simulink model "cartpole"  (R2016a)
settings: Solver=ode23s  StartTime=0.0  StopTime=90  RelTol=1e-3
values from neighbouring files (symbols this model uses):
  g = 9.81    [cartPole.mat]
  K = lqr(A,B,Q,R)    [KDC_HW2_Problem4_LQR.m]    (also in cartPole.mat = [143.360926463 -1 35.2365734727 -11.2706480711])
  kd = 0.1    [cartPole.mat]
  ke = 2    [cartPole.mat]
  kp = 0.1    [cartPole.mat]
  l = 1    [cartPole.mat]
  mc = 1    [cartPole.mat]
  mp = 0.1    [cartPole.mat]
libraries: mblibv1 x11, simulink x1
settings Model: Creator=Bradley Factor  LastModifiedBy=Bradley Factor
settings SolverCC: MaxConsecutiveMinStep=100
settings SimMechanicsCC: VisDuringSimulation=on

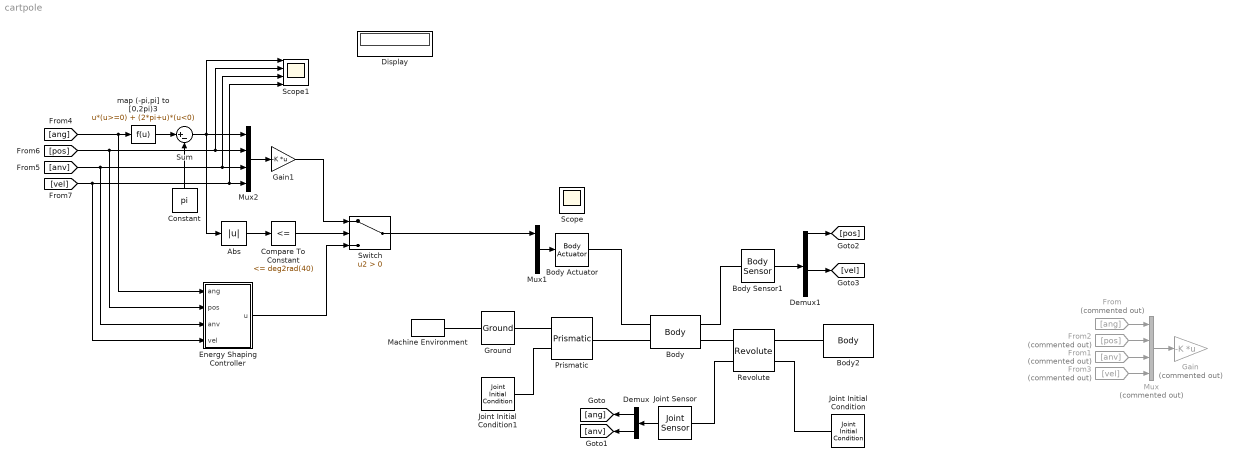
== system cartpole ==
  Abs : Abs
  Body : mblibv1/Bodies/Body  LConnTagsString=CS4|CS1  RConnTagsString=CG|CS3  UpdateFromCAD=off  DialogClass=MechanicalBodyBlock  Mass=1  MassUnits=kg  InertiaUnits=kg*m^2  Inertia=eye(3)  Shape=Cylinder  ShapeDims=[1 1]  ShapeUnits=m  ShapeUse=false  Density=1  DensityUnits=kg/m^3  DensityUse=false  GraphicsMode=MACHINE_DEFAULT  BodyColorSelMode=MACHINE_DEFAULT  BodyColor=[1 0 0]  AttachedToCS=CG  CG=Right$CG$[0.25 0 0]$CS1$CS1$m$[0 0 0]$Euler X-Y-Z$deg$WORLD$true$none  WorkingFrames=Left$CS4$[0 0 0]$CG$CG$m$[0 0 0]$Euler X-Y-Z$deg$WORLD$true$none#Left$CS1$[-0.25 0 0]$Adjoining$Adjoining$m$[0 0 0]$Euler X-Y-Z$deg$WORLD$true$none#Right$CS2$[0.5 0 0]$CS1$CS1$m$[0 0 0]$Euler X-Y-Z$deg$WORLD$false$none#Right$CS3$[0 0 0]$CG$CG$m$[0 0 0]$Euler X-Y-Z$deg$WORLD$true$none  CGPos=[0.25 0 0]  CGRot=[0 0 0]  CS0Pos=[]  CS0Rot=[]  CS1Pos=[-0.25 0 0]  CS1Rot=[0 0 0]  CS2Pos=[0.5 0 0]  CS2Rot=[0 0 0]  CS3Pos=[0 0 0]  CS3Rot=[0 0 0]  CS4Pos=[0 0 0]  CS4Rot=[0 0 0]  CS5Pos=[]  CS5Rot=[]  CS6Pos=[]  CS6Rot=[]  CS7Pos=[]  CS7Rot=[]  CS8Pos=[]  CS8Rot=[]  CS9Pos=[]  CS9Rot=[]  CS10Pos=[]  CS10Rot=[]  CS11Pos=[]  CS11Rot=[]  CS12Pos=[]  CS12Rot=[]  CS13Pos=[]  CS13Rot=[]  CS14Pos=[]  CS14Rot=[]  CS15Pos=[]  CS15Rot=[]  CS16Pos=[]  CS16Rot=[]  CS17Pos=[]  CS17Rot=[]  CS18Pos=[]  CS18Rot=[]  CS19Pos=[]  CS19Rot=[]  CS20Pos=[]  CS20Rot=[]
  Body Actuator : mblibv1/Sensors &  Actuators/Body Actuator  UpdateFromCAD=off  PhysicalDomain=Mechanical  PortType=blob  ActuationStyle=Force  AngleUnits=deg  ArcVelocityUnits=deg/s  ArcAccelerationUnits=deg/s^2  CoordPositionUnits=m  VelocityUnits=m/s  AccelerationUnits=m/s^2  ForceUnits=N  TorqueUnits=N-m  ActiveIO=on  Width=3  DialogClass=MechanicalActuatorBlock  ReferenceFrame=Absolute (World)  Angle=off  CoordPosition=on  Force=on  Torque=off
  Body Sensor1 : mblibv1/Sensors &  Actuators/Body Sensor  UpdateFromCAD=off  PhysicalDomain=Mechanical  PortType=blob  Muxed=on  Pose=off  Angle=on  AngleUnits=deg  ArcVelocity=off  ArcVelocityUnits=deg/s  ArcAcceleration=off  ArcAccelerationUnits=deg/s^2  CoordPosition=on  CoordPositionUnits=m  Velocity=on  VelocityUnits=m/s  Acceleration=off  AccelerationUnits=m/s^2  Quaternion=on  QuaternionDT=off  QuaternionDDT=off  QuaternionUnits=off  OutputVector=[1]  ActiveIO=on  Width=6  DialogClass=MechanicalSensorBlock  ReferenceFrame=Absolute (World)
  Body2 : mblibv1/Bodies/Body  LConnTagsString=CS1  UpdateFromCAD=off  DialogClass=MechanicalBodyBlock  Mass=0.1  MassUnits=kg  InertiaUnits=kg*m^2  Inertia=[1/3*0.1*1 0 0; 0 0 0; 0 0 1/3*0.1*1]  Shape=Cylinder  ShapeDims=[1 1]  ShapeUnits=m  ShapeUse=false  Density=1  DensityUnits=kg/m^3  DensityUse=false  GraphicsMode=MACHINE_DEFAULT  BodyColorSelMode=MACHINE_DEFAULT  BodyColor=[1 0 0]  AttachedToCS=CG  CG=Left$CG$[0 -0.5 0]$CS1$CS1$m$[0 0 0]$Euler X-Y-Z$deg$WORLD$false$none  WorkingFrames=Left$CS1$[0 0 0]$Adjoining$Adjoining$m$[0 0 0]$Euler X-Y-Z$deg$WORLD$true$none#Right$CS2$[0 -1 0]$CS1$CS1$m$[0 0 0]$Euler X-Y-Z$deg$WORLD$false$none  CGPos=[0 -0.5 0]  CGRot=[0 0 0]  CS0Pos=[]  CS0Rot=[]  CS1Pos=[0 0 0]  CS1Rot=[0 0 0]  CS2Pos=[0 -1 0]  CS2Rot=[0 0 0]  CS3Pos=[]  CS3Rot=[]  CS4Pos=[]  CS4Rot=[]  CS5Pos=[]  CS5Rot=[]  CS6Pos=[]  CS6Rot=[]  CS7Pos=[]  CS7Rot=[]  CS8Pos=[]  CS8Rot=[]  CS9Pos=[]  CS9Rot=[]  CS10Pos=[]  CS10Rot=[]  CS11Pos=[]  CS11Rot=[]  CS12Pos=[]  CS12Rot=[]  CS13Pos=[]  CS13Rot=[]  CS14Pos=[]  CS14Rot=[]  CS15Pos=[]  CS15Rot=[]  CS16Pos=[]  CS16Rot=[]  CS17Pos=[]  CS17Rot=[]  CS18Pos=[]  CS18Rot=[]  CS19Pos=[]  CS19Rot=[]  CS20Pos=[]  CS20Rot=[]
  Compare To Constant : simulink/Logic and Bit Operations/Compare To Constant  relop=<=  const=deg2rad(40)  OutDataTypeStr=boolean
  Constant : Constant  Value=pi
  Demux : Demux  Outputs=2
  Demux1 : Demux  Outputs=6
  Display : Display
  Energy Shaping Controller : Subsystem
  From : From  Commented=on  GotoTag=ang
  From1 : From  Commented=on  GotoTag=anv
  From2 : From  Commented=on  GotoTag=pos
  From3 : From  Commented=on  GotoTag=vel
  Gain : Gain  Commented=on  Gain=-K  Multiplication=Matrix(K*u)
  Gain1 : Gain  Gain=-K  Multiplication=Matrix(K*u)
  Ground : mblibv1/Bodies/Ground  UpdateFromCAD=off  LeftPortType=env  RightPortType=workingframe  PhysicalDomain=Mechanical  DialogClass=GroundBlock  CoordPosition=[0 0 0]  CoordPositionUnits=m  StateVectorMgrId=0  MachineId=[1 0]  ShowEnvPort=on  ParameterChecksum=[3037818671, 2405939126, 2614509267, 208361322]  TopologyChecksum=[3963185961, 293394640, 1509995164, 4077453628]
  Joint Initial Condition : mblibv1/Sensors &  Actuators/Joint Initial Condition  UpdateFromCAD=off  LeftPortType=blob  RightPortType=blob  PhysicalDomain=mechanical  DialogClass=InitialConditionBlock  InitialConditions=P1$false$0$m$deg$0$m/s$deg/s#P2$false$0$m$deg$0$m/s$deg/s#P3$false$0$m$deg$0$m/s$deg/s#R1$true$deg2rad(10)$m$rad$deg2rad(0)$m/s$rad/s#R2$false$0$m$deg$0$m/s$deg/s#R3$false$0$m$deg$0$m/s$deg/s#S$false$0$m$deg$0$m/s$deg/s  P1PIC=0  P1VIC=0  P2PIC=0  P2VIC=0  P3PIC=0  P3VIC=0  R1PIC=deg2rad(10)  R1VIC=deg2rad(0)  R2PIC=0  R2VIC=0  R3PIC=0  R3VIC=0  SPIC=0  SVIC=0
  Joint Initial Condition1 : mblibv1/Sensors &  Actuators/Joint Initial Condition  UpdateFromCAD=off  LeftPortType=blob  RightPortType=blob  PhysicalDomain=mechanical  DialogClass=InitialConditionBlock  InitialConditions=P1$true$0$m$deg$0$m/s$deg/s#P2$false$0$m$deg$0$m/s$deg/s#P3$false$0$m$deg$0$m/s$deg/s#R1$false$0$m$deg$0$m/s$deg/s#R2$false$0$m$deg$0$m/s$deg/s#R3$false$0$m$deg$0$m/s$deg/s#S$false$0$m$deg$0$m/s$deg/s  P1PIC=0  P1VIC=0  P2PIC=0  P2VIC=0  P3PIC=0  P3VIC=0  R1PIC=0  R1VIC=0  R2PIC=0  R2VIC=0  R3PIC=0  R3VIC=0  SPIC=0  SVIC=0
  Joint Sensor : mblibv1/Sensors &  Actuators/Joint Sensor  UpdateFromCAD=off  PhysicalDomain=Mechanical  PortType=blob  Muxed=on  Pose=off  Angle=on  AngleUnits=rad  ArcVelocity=on  ArcVelocityUnits=rad/s  ArcAcceleration=off  ArcAccelerationUnits=deg/s^2  CoordPosition=on  CoordPositionUnits=m  Velocity=off  VelocityUnits=m/s  Acceleration=off  AccelerationUnits=m/s^2  Quaternion=on  QuaternionDT=off  QuaternionDDT=off  QuaternionUnits=off  OutputVector=[1]  ActiveIO=on  Width=2  DialogClass=MechanicalSensorBlock  Primitive=R1  Force=off  ForceUnits=N  Torque=off  TorqueUnits=N*m  ReferenceFrame=Absolute (World)  ReactionSensedSide=Base  ReactionReferenceFrame=Absolute (World)  ReactionForce=off  ReactionForceUnits=N  ReactionMoment=off  ReactionMomentUnits=N*m
  Machine Environment : mblibv1/Bodies/Machine Environment  PortType=env  PhysicalDomain=Mechanical  DialogTemplateClass=MECH.MachineEnvironment  SyncWhenCopied=off  Gravity=[0 -9.81 0]  GravityUnits=m/s^2  GravityAsSignal=off  Dimensionality=Auto-detect  AnalysisType=Forward dynamics  LinearAssemblyTolerance=1e-3  LinearAssemblyToleranceUnits=m  AngularAssemblyTolerance=1e-3  AngularAssemblyToleranceUnits=rad  ConstraintSolverType=Stabilizing  ConstraintRelTolerance=1e-4  ConstraintAbsTolerance=1e-4  UseRobustSingularityHandling=off  RedundancyAnalysisToleranceType=Automatically select tolerance  RedundancyAnalysisTolerance=1e-14  StatePerturbationType=Fixed  PerturbationSize=1e-5  VisualizeMachine=on  BodyVisualizationType=Use model default body geometries  BodyColorSelMode=Use model default  DefaultBodyColor=[1 0 0]
  Mux : Mux  Commented=on
  Mux1 : Mux  Inputs=3
  Mux2 : Mux
  Prismatic : mblibv1/Joints/Prismatic  LConnTagsString=__newl0|SA1  RConnTagsString=__newr0  UpdateFromCAD=off  NumSAPorts=1  CutJoint=off  MarkAsCut=off  Primitives=prismatic  PrimitiveProps=P1$World$[1 0 0]$prismatic  DialogClass=JointBlock  P1Axis=[1 0 0]
  Revolute : mblibv1/Joints/Revolute  LConnTagsString=__newl0|SA1  RConnTagsString=__newr0|SA1  UpdateFromCAD=off  NumSAPorts=2  CutJoint=off  MarkAsCut=off  Primitives=prismatic  PrimitiveProps=R1$Base$[0 0 1]$revolute  DialogClass=JointBlock  R1Axis=[0 0 1]
  Scope : Scope
  Scope1 : Scope  NumInputPorts=4
  Sum : Sum  Inputs=|+-
  Switch : Switch  Criteria=u2 > Threshold
  map (-pi,pi] to [0,2pi)3 : Fcn  Expr=u*(u>=0) + (2*pi+u)*(u<0)
  wires:
  Joint Sensor/1 -> Demux/1
  Demux/1 -> [ang]
  Demux/2 -> [anv]
  Body Sensor1/1 -> Demux1/1
  Demux1/1 -> [pos]
  Mux1/1 -> Body Actuator/1
  Demux1/4 -> [vel]
  Mux/1 -> Gain/1
  From1/1 -> Mux/3
  From3/1 -> Mux/4
  From2/1 -> Mux/2
  From/1 -> Mux/1
  [anv] -> Energy Shaping Controller/3(anv), Mux2/3, Scope1/3
  [vel] -> Energy Shaping Controller/4(vel), Mux2/4, Scope1/4
  [pos] -> Energy Shaping Controller/2(pos), Mux2/2, Scope1/2
  Mux2/1 -> Gain1/1
  [ang] -> Energy Shaping Controller/1(ang), map (-pi,pi] to [0,2pi)3/1
  map (-pi,pi] to [0,2pi)3/1 -> Sum/1
  Sum/1 -> Abs/1, Scope1/1, Mux2/1
  Constant/1 -> Sum/2
  Abs/1 -> Compare To Constant/1
  Compare To Constant/1 -> Switch/2
  Gain1/1 -> Switch/1
  Switch/1 -> Mux1/1
  Energy Shaping Controller/1(u) -> Switch/3
  connections:
  Machine Environment/RConn1 -- Ground/LConn1
  Prismatic/LConn1 -- Ground/RConn1
  Body2/LConn1 -- Revolute/RConn1
  Joint Initial Condition/RConn1 -- Revolute/RConn2
  Joint Initial Condition1/RConn1 -- Prismatic/LConn2
  Prismatic/RConn1 -- Body/LConn2
  Body/RConn2 -- Revolute/LConn1
  Body Actuator/RConn1 -- Body/LConn1
  Body Sensor1/LConn1 -- Body/RConn1
  Joint Sensor/LConn1 -- Revolute/LConn2

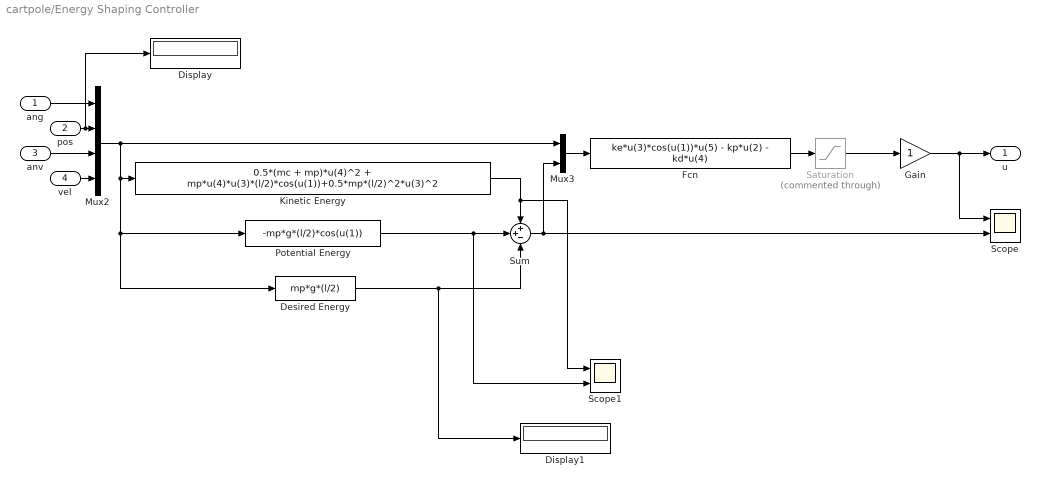
== system cartpole/Energy Shaping Controller ==
  ang : Inport
  pos : Inport  Port=2
  anv : Inport  Port=3
  vel : Inport  Port=4
  Desired Energy : Fcn  Expr=mp*g*(l/2)
  Display : Display
  Display1 : Display
  Fcn : Fcn  Expr=ke*u(3)*cos(u(1))*u(5) - kp*u(2) - kd*u(4)
  Gain : Gain
  Kinetic Energy : Fcn  Expr=0.5*(mc + mp)*u(4)^2 + mp*u(4)*u(3)*(l/2)*cos(u(1))+0.5*mp*(l/2)^2*u(3)^2
  Mux2 : Mux
  Mux3 : Mux  Inputs=2
  Potential Energy : Fcn  Expr=-mp*g*(l/2)*cos(u(1))
  Saturation : Saturate  Commented=through  UpperLimit=1e6  LowerLimit=-1e6
  Scope : Scope  NumInputPorts=2
  Scope1 : Scope  NumInputPorts=2
  Sum : Sum  Inputs=++-
  u : Outport
  wires:
  Sum/1 -> Mux3/2, Scope/2
  Mux2/1 -> Potential Energy/1, Desired Energy/1, Kinetic Energy/1, Mux3/1
  pos/1 -> Display/1, Mux2/2
  anv/1 -> Mux2/3
  vel/1 -> Mux2/4
  ang/1 -> Mux2/1
  Mux3/1 -> Fcn/1
  Fcn/1 -> Saturation/1
  Saturation/1 -> Gain/1
  Kinetic Energy/1 -> Scope1/1, Sum/1
  Potential Energy/1 -> Scope1/2, Sum/2
  Desired Energy/1 -> Display1/1, Sum/3
  Gain/1 -> Scope/1, u/1
